simulink subsystem "Zustandsregler"  (R2020a)
settings: Solver=VariableStepAuto  StartTime=0.0  StopTime=10.0  RelTol=1e-3
model mask{K=[], xtype=Zustandsmessung, beob=[]}
  mask prompts: xtype "Zustandsermittlung"; beob "Beobachter"
values from neighbouring files (symbols this model uses):
  L = place(sys.A', sys.C', pole).'    [PlaceBeobachter.m]
undefined symbols (not defined in the file or in its folder): A, B, C
libraries: dspfdesign x3
settings Model: Creator=Tobias  LastModifiedBy=Tobias

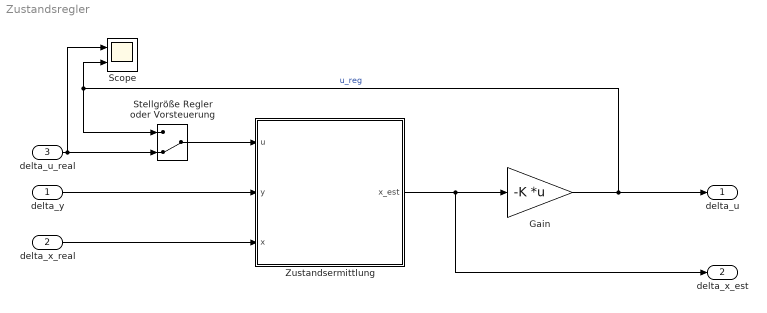
== system Zustandsregler ==
  delta_y : Inport
  delta_x_real : Inport  Port=2
  delta_u_real : Inport  Port=3
  Gain : Gain  Gain=-K  Multiplication=Matrix(K*u)
  Scope : Scope  NumInputPorts=2
  Stellgröße Regler oder Vorsteuerung : ManualSwitch  CurrentSetting=0
  Zustandsermittlung : Subsystem  Variant=on  VariantControl=Choice  PropagateVariantConditions=on
  delta_u : Outport
  delta_x_est : Outport  Port=2
  wires:
  delta_x_real/1 -> Zustandsermittlung/3(x)
  Zustandsermittlung/1(x_est) -> Gain/1, delta_x_est/1
  delta_y/1 -> Zustandsermittlung/2(y)
  Gain/1 -> delta_u/1, Stellgröße Regler oder Vorsteuerung/1, Scope/2  "u_reg"
  Stellgröße Regler oder Vorsteuerung/1 -> Zustandsermittlung/1(u)
  delta_u_real/1 -> Scope/1, Stellgröße Regler oder Vorsteuerung/2

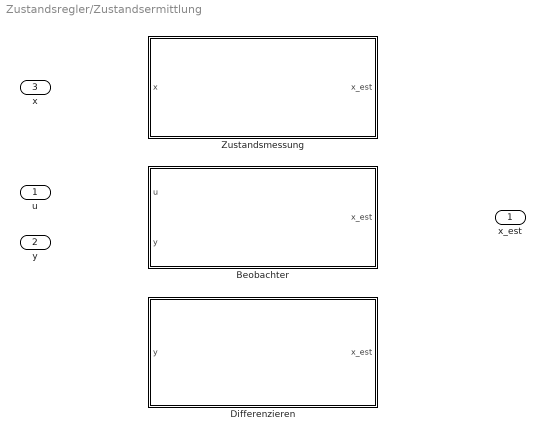
== system Zustandsregler/Zustandsermittlung ==
  u : Inport
  y : Inport  Port=2
  x : Inport  Port=3
  Beobachter : Subsystem  VariantControl=simparams.Zustandsermittlung==2
  Differenzieren : Subsystem  VariantControl=simparams.Zustandsermittlung==3
  Zustandsmessung : Subsystem  VariantControl=simparams.Zustandsermittlung==1
  x_est : Outport

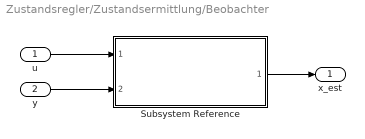
== system Zustandsregler/Zustandsermittlung/Beobachter ==
  u : Inport
  y : Inport  Port=2
  Subsystem Reference : Subsystem  ReferencedSubsystem=Beobachter  A=A  B=B  C=C  L=L  xb0=xb0
  x_est : Outport
  wires:
  Subsystem Reference/1 -> x_est/1
  y/1 -> Subsystem Reference/2
  u/1 -> Subsystem Reference/1

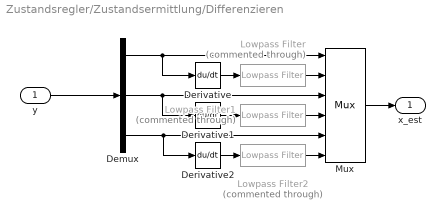
== system Zustandsregler/Zustandsermittlung/Differenzieren ==
  y : Inport
  Demux : Demux  Outputs=3
  Derivative : Derivative  CoefficientInTFapproximation=1
  Derivative1 : Derivative  CoefficientInTFapproximation=1
  Derivative2 : Derivative  CoefficientInTFapproximation=1
  Lowpass Filter : dspfdesign/Lowpass Filter  Commented=through  FilterType=FIR  DesignForMinimumOrder=on  FilterOrder=50  PassbandFrequency=25  StopbandFrequency=100  PassbandRipple=0.1  StopbandAttenuation=80  InheritSampleRate=off  SampleRate=1000  SimulateUsing=Interpreted execution  roundingMode=Floor  coeffsDataTypeStr=fixdt(1,16)
  Lowpass Filter1 : dspfdesign/Lowpass Filter  Commented=through  FilterType=FIR  DesignForMinimumOrder=on  FilterOrder=50  PassbandFrequency=25  StopbandFrequency=100  PassbandRipple=0.1  StopbandAttenuation=80  InheritSampleRate=off  SampleRate=1000  SimulateUsing=Interpreted execution  roundingMode=Floor  coeffsDataTypeStr=fixdt(1,16)
  Lowpass Filter2 : dspfdesign/Lowpass Filter  Commented=through  FilterType=FIR  DesignForMinimumOrder=on  FilterOrder=50  PassbandFrequency=25  StopbandFrequency=100  PassbandRipple=0.1  StopbandAttenuation=80  InheritSampleRate=off  SampleRate=1000  SimulateUsing=Interpreted execution  roundingMode=Floor  coeffsDataTypeStr=fixdt(1,16)
  Mux : Mux  Inputs=6
  x_est : Outport
  wires:
  Mux/1 -> x_est/1
  y/1 -> Demux/1
  Demux/1 -> Derivative/1, Mux/1
  Demux/2 -> Derivative1/1, Mux/3
  Demux/3 -> Derivative2/1, Mux/5
  Derivative/1 -> Lowpass Filter/1
  Derivative1/1 -> Lowpass Filter1/1
  Derivative2/1 -> Lowpass Filter2/1
  Lowpass Filter/1 -> Mux/2
  Lowpass Filter1/1 -> Mux/4
  Lowpass Filter2/1 -> Mux/6

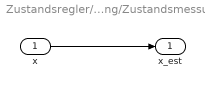
== system Zustandsregler/Zustandsermittlung/Zustandsmessung ==
  x : Inport
  x_est : Outport
  wires:
  x/1 -> x_est/1
